simulink model "chap1_7sim"  (R2019a)
settings: Solver=VariableStepAuto  StartTime=0.0  StopTime=10.0  RelTol=1e-3
settings Model: Creator=smilingfrog  LastModifiedBy=smilingfrog
settings DataIOCC: ReturnWorkspaceOutputs=off

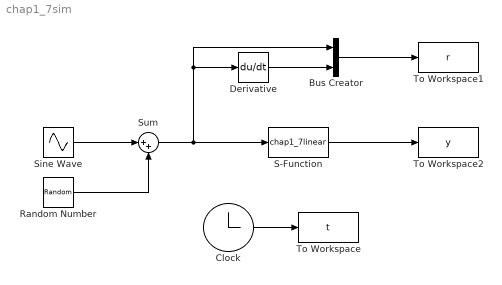
== system chap1_7sim ==
  Bus Creator : BusCreator  Inputs=2
  Clock : Clock
  Derivative : Derivative
  Random Number : RandomNumber  Variance=0.1  SampleTime=0.001
  S-Function : S-Function  FunctionName=chap1_7linear  SFunctionDeploymentMode=off  EnableBusSupport=off
  Sine Wave : Sin  SampleTime=0
  Sum : Sum  Inputs=|++
  To Workspace : ToWorkspace  VariableName=t  SampleTime=-1
  To Workspace1 : ToWorkspace  VariableName=r  SampleTime=-1
  To Workspace2 : ToWorkspace  VariableName=y  SampleTime=-1
  wires:
  Sine Wave/1 -> Sum/1
  Derivative/1 -> Bus Creator/2
  Random Number/1 -> Sum/2
  Sum/1 -> Bus Creator/1, Derivative/1, S-Function/1
  Clock/1 -> To Workspace/1
  S-Function/1 -> To Workspace2/1
  Bus Creator/1 -> To Workspace1/1
